simulink subsystem "Modelo_R2023b"  (R2023b)
settings: Solver=VariableStepAuto  StartTime=0.0  StopTime=10.0  RelTol=1e-3
values from neighbouring files (symbols this model uses):
  alpha_Cu = 3.9e-3    (= 0.0039)    [coeficientes.m]
  b_eq = b_m + b_l/(r_m2l^2)    (= 2.19444444444e-05)    [coeficientes.m]
  C_ts = 0.818    [coeficientes.m]
  g = 9.80665    [coeficientes.m]
  J_eq = J_m + J_l/(r_m2l^2)    (= 4.58263888889e-05)    [coeficientes.m]
  k_l = 0.1    [coeficientes.m]
  L_d = 6.6e-3    (= 0.0066)    [coeficientes.m]
  L_ls = 0.8e-3    (= 0.0008)    [coeficientes.m]
  L_q = 5.8e-3    (= 0.0058)    [coeficientes.m]
  lambda = 0.016    [coeficientes.m]
  Pp = 3    [coeficientes.m]
  r_m2l = 120.0    (= 120)    [coeficientes.m]
  R_sREF = 1.02    [coeficientes.m]
  R_tsamb = 146.7    [coeficientes.m]
  T_amb = 20    [coeficientes.m]
  T_sREF = 20    [coeficientes.m]
libraries: mcbcontrolslib x2
settings Model: Creator=barrios14101  LastModifiedBy=barrios14101
settings RTWCC: GPUComputeCapability=5.0
settings ConfigComp: CovBoundaryAbsTol=1.0e-5

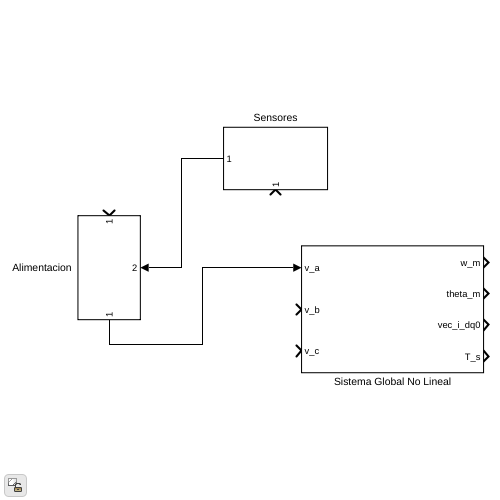
[thumbnail: Simulink's stored preview of the top-level diagram]
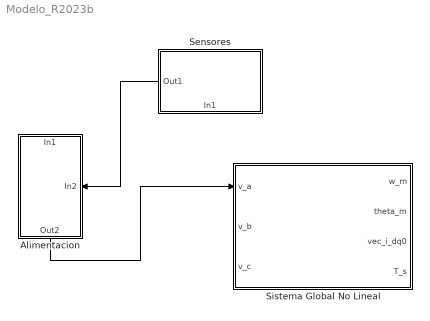
== system Modelo_R2023b ==
  Alimentacion : Subsystem
      settings: PortSchema="{\"entries\":[{\"content\":{\"sides\":[{\"content\":{\"connectorIds\":[\"In1\"]},\"type\":\"ConnectorPlacement.EquallySpacedRectSide\",\"uuid\":\"0c953847-a542-44e1-afa1-eb16e3fe163f\"},{\"content\":{\"connectorIds\":[\"Out1\"],\"side\":\"RIGHT\"},\"type\":\"ConnectorPlacement.EquallySpacedRectSide\",\"uuid\":\"d6f8d29b-16c5-463f-b013-7003ed613fe0\"},{\"content\":{\"connectorIds\":[\"In2\"],\"side\":\"TOP\"},\"type\":\"ConnectorPlacement.EquallySpacedRectSide\",\"uuid\":\"60c3fb2f-c7a9-4bb3-be2b-510700c2fe0f\"},{\"content\":{\"side\":\"BOTTOM\"},\"type\":\"ConnectorPlacement.EquallySpacedRectSide\",\"uuid\":\"5571030c-c37f-4b87-b6e8-9288f1bd1f58\"}]},\"type\":\"ConnectorPlacement.EquallySpacedConnector\",\"uuid\":\"8bfbadc8-fb17-4150-9925-c98e8d49e11f\"}],\"packageUris\":[\"http://schema.mathworks.com/mf0/Connector/R2020b\"],\"version\":\"1.0\"}"
  Sensores : Subsystem
      settings: PortSchema="{\"entries\":[{\"content\":{\"sides\":[{\"content\":{\"connectorIds\":[\"Out1\"]},\"type\":\"ConnectorPlacement.EquallySpacedRectSide\",\"uuid\":\"0c953847-a542-44e1-afa1-eb16e3fe163f\"},{\"content\":{\"side\":\"RIGHT\"},\"type\":\"ConnectorPlacement.EquallySpacedRectSide\",\"uuid\":\"d6f8d29b-16c5-463f-b013-7003ed613fe0\"},{\"content\":{\"side\":\"TOP\"},\"type\":\"ConnectorPlacement.EquallySpacedRectSide\",\"uuid\":\"60c3fb2f-c7a9-4bb3-be2b-510700c2fe0f\"},{\"content\":{\"connectorIds\":[\"In1\"],\"side\":\"BOTTOM\"},\"type\":\"ConnectorPlacement.EquallySpacedRectSide\",\"uuid\":\"48731a4e-21f3-48a9-965b-1bc0b841acdd\"}]},\"type\":\"ConnectorPlacement.EquallySpacedConnector\",\"uuid\":\"8bfbadc8-fb17-4150-9925-c98e8d49e11f\"}],\"packageUris\":[\"http://schema.mathworks.com/mf0/Connector/R2020b\"],\"version\":\"1.0\"}"
  Sistema Global No Lineal : Subsystem
  wires:
  Alimentacion/1(Out2) -> Sistema Global No Lineal/1(v_a)
  Sensores/1(Out1) -> Alimentacion/2(In2)

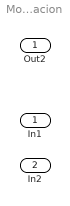
== system Modelo_R2023b/Alimentacion ==
  In1 : Inport
  In2 : Inport  Port=2
  Out2 : Outport

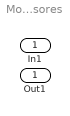
== system Modelo_R2023b/Sensores ==
  In1 : Inport
  Out1 : Outport

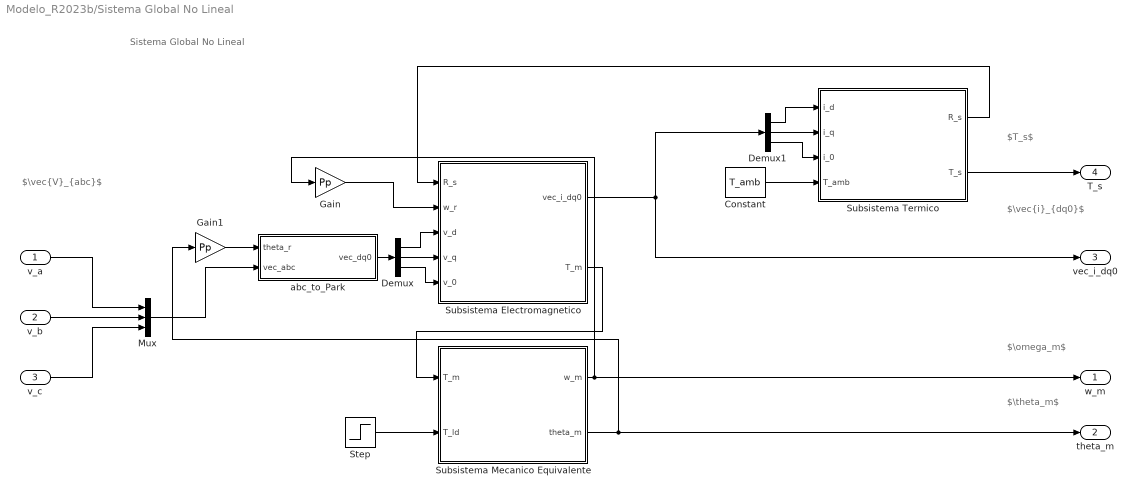
== system Modelo_R2023b/Sistema Global No Lineal ==
  note: $\omega_m$
  note: $T_s$
  note: $\vec{i}_{dq0}$
  note: $\vec{V}_{abc}$
  note: Sistema Global No Lineal
  note: $\theta_m$
  v_a : Inport
  v_b : Inport  Port=2
  v_c : Inport  Port=3
  Constant : Constant  Value=T_amb
  Demux : Demux  Outputs=3
  Demux1 : Demux  Outputs=3
  Gain : Gain  Gain=Pp
  Gain1 : Gain  Gain=Pp
  Mux : Mux  Inputs=3
  Step : Step  Time=0  After=15  SampleTime=0
  Subsistema Electromagnetico : Subsystem
  Subsistema Mecanico Equivalente : Subsystem
  Subsistema Termico : Subsystem
  abc_to_Park : Subsystem  TreatAsAtomicUnit=on
  w_m : Outport
  theta_m : Outport  Port=2
  vec_i_dq0 : Outport  Port=3
  T_s : Outport  Port=4
  wires:
  Subsistema Termico/2(T_s) -> T_s/1
  Subsistema Electromagnetico/1(vec_i_dq0) -> vec_i_dq0/1, Demux1/1
  Subsistema Mecanico Equivalente/1(w_m) -> w_m/1, Gain/1
  Subsistema Mecanico Equivalente/2(theta_m) -> theta_m/1, Gain1/1
  Subsistema Electromagnetico/2(T_m) -> Subsistema Mecanico Equivalente/1(T_m)
  Demux1/2 -> Subsistema Termico/2(i_q)
  Subsistema Termico/1(R_s) -> Subsistema Electromagnetico/1(R_s)
  abc_to_Park/1(vec_dq0) -> Demux/1
  Gain1/1 -> abc_to_Park/1(theta_r)
  Gain/1 -> Subsistema Electromagnetico/2(w_r)
  Step/1 -> Subsistema Mecanico Equivalente/2(T_ld)
  v_a/1 -> Mux/1
  Mux/1 -> abc_to_Park/2(vec_abc)
  Demux1/1 -> Subsistema Termico/1(i_d)
  v_b/1 -> Mux/2
  Demux/3 -> Subsistema Electromagnetico/5(v_0)
  Demux/2 -> Subsistema Electromagnetico/4(v_q)
  Demux/1 -> Subsistema Electromagnetico/3(v_d)
  Demux1/3 -> Subsistema Termico/3(i_0)
  v_c/1 -> Mux/3
  Constant/1 -> Subsistema Termico/4(T_amb)

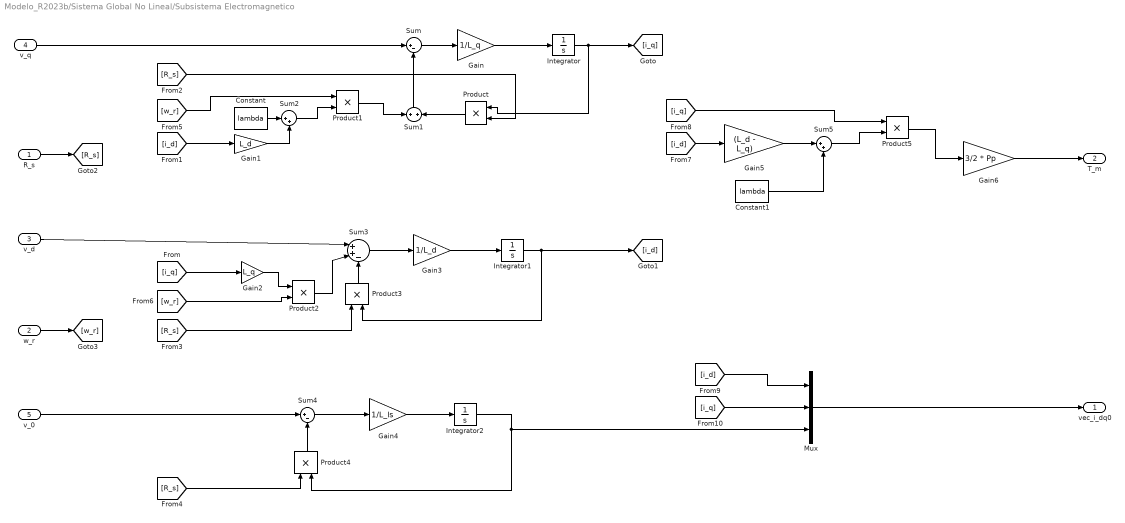
== system Modelo_R2023b/Sistema Global No Lineal/Subsistema Electromagnetico ==
  R_s : Inport
  w_r : Inport  Port=2
  v_d : Inport  Port=3
  v_q : Inport  Port=4
  v_0 : Inport  Port=5
  Constant : Constant  Value=lambda
  Constant1 : Constant  Value=lambda
  Gain : Gain  Gain=1/L_q
  Gain1 : Gain  Gain=L_d
  Gain2 : Gain  Gain=L_q
  Gain3 : Gain  Gain=1/L_d
  Gain4 : Gain  Gain=1/L_ls
  Gain5 : Gain  Gain=(L_d - L_q)
  Gain6 : Gain  Gain=3/2 * Pp
  Integrator : Integrator
  Integrator1 : Integrator
  Integrator2 : Integrator
  Mux : Mux  Inputs=3
  Product{,1..5} (6 alike) : Product
  Sum : Sum  Inputs=|+-
  Sum1 : Sum
  Sum2 : Sum  Inputs=|++
  Sum3 : Sum  Inputs=|++-
  Sum4 : Sum  Inputs=|+-
  Sum5 : Sum  Inputs=|++
  vec_i_dq0 : Outport
  T_m : Outport  Port=2
  wires:
  Gain1/1 -> Sum2/2
  Product1/1 -> Sum1/1
  Sum2/1 -> Product1/2
  Constant/1 -> Sum2/1
  Product/1 -> Sum1/2
  Sum/1 -> Gain/1
  Sum1/1 -> Sum/2
  v_q/1 -> Sum/1
  Gain/1 -> Integrator/1
  Product3/1 -> Sum3/3
  Gain3/1 -> Integrator1/1
  Sum3/1 -> Gain3/1
  Product2/1 -> Sum3/2
  Gain2/1 -> Product2/1
  v_d/1 -> Sum3/1
  Product4/1 -> Sum4/2
  Integrator2/1 -> Mux/3, Product4/2
  Gain4/1 -> Integrator2/1
  Sum4/1 -> Gain4/1
  v_0/1 -> Sum4/1
  Gain5/1 -> Sum5/1
  Sum5/1 -> Product5/2
  Integrator1/1 -> [i_d], Product3/2
  Constant1/1 -> Sum5/2
  Product5/1 -> Gain6/1
  Integrator/1 -> [i_q], Product/1
  Gain6/1 -> T_m/1
  [i_q] -> Gain2/1
  [i_d] -> Gain1/1
  [R_s] -> Product/2
  R_s/1 -> [R_s]
  [R_s] -> Product3/1
  [R_s] -> Product4/1
  w_r/1 -> [w_r]
  [w_r] -> Product1/1
  [w_r] -> Product2/2
  [i_d] -> Gain5/1
  [i_q] -> Product5/1
  [i_q] -> Mux/2
  [i_d] -> Mux/1
  Mux/1 -> vec_i_dq0/1

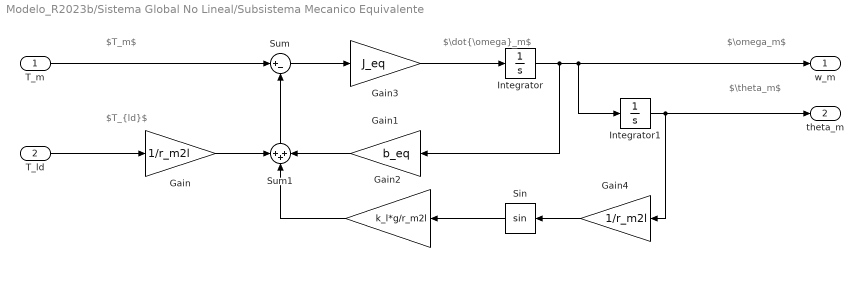
== system Modelo_R2023b/Sistema Global No Lineal/Subsistema Mecanico Equivalente ==
  note: $T_m$
  note: $T_{ld}$
  note: $\dot{\omega}_m$
  note: $\omega_m$
  note: $\theta_m$
  T_m : Inport
  T_ld : Inport  Port=2
  Gain : Gain  Gain=1/r_m2l
  Gain1 : Gain  Gain=b_eq
  Gain2 : Gain  Gain=k_l*g/r_m2l
  Gain3 : Gain  Gain=J_eq
  Gain4 : Gain  Gain=1/r_m2l
  Integrator : Integrator
  Integrator1 : Integrator
  Sin : Trigonometry
  Sum : Sum  Inputs=|+-
  Sum1 : Sum  Inputs=+++
  w_m : Outport
  theta_m : Outport  Port=2
  wires:
  Integrator/1 -> Integrator1/1, w_m/1, Gain1/1
  Integrator1/1 -> theta_m/1, Gain4/1
  Sum/1 -> Gain3/1
  T_m/1 -> Sum/1
  Sum1/1 -> Sum/2
  Gain2/1 -> Sum1/2
  Gain/1 -> Sum1/1
  Sin/1 -> Gain2/1
  Gain1/1 -> Sum1/3
  Gain3/1 -> Integrator/1
  Gain4/1 -> Sin/1
  T_ld/1 -> Gain/1

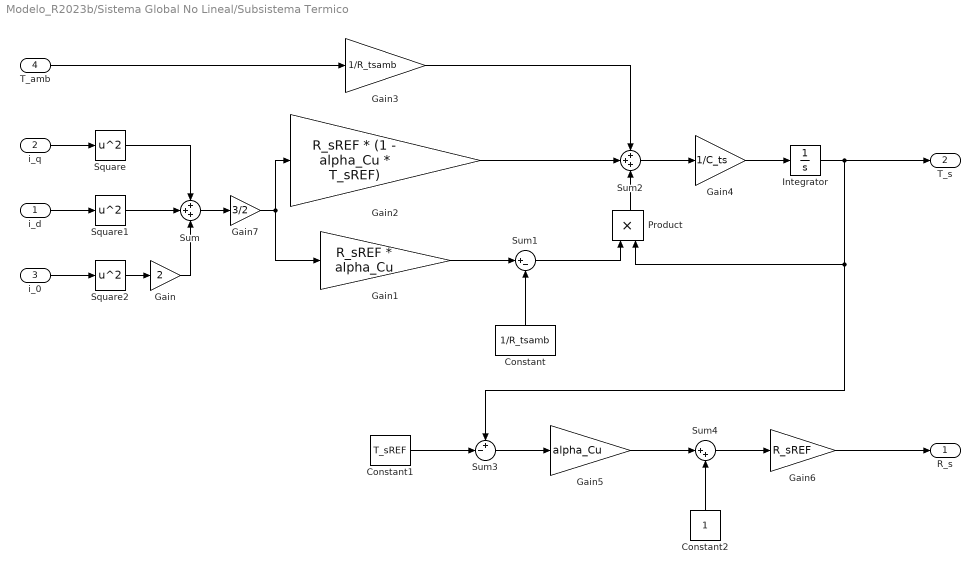
== system Modelo_R2023b/Sistema Global No Lineal/Subsistema Termico ==
  i_d : Inport
  i_q : Inport  Port=2
  i_0 : Inport  Port=3
  T_amb : Inport  Port=4
  Constant : Constant  Value=1/R_tsamb
  Constant1 : Constant  Value=T_sREF
  Constant2 : Constant
  Gain : Gain  Gain=2
  Gain1 : Gain  Gain=R_sREF * alpha_Cu
  Gain2 : Gain  Gain="R_sREF * (1 -  alpha_Cu * T_sREF)"
  Gain3 : Gain  Gain=1/R_tsamb
  Gain4 : Gain  Gain=1/C_ts
  Gain5 : Gain  Gain=alpha_Cu
  Gain6 : Gain  Gain=R_sREF
  Gain7 : Gain  Gain=3/2
  Integrator : Integrator
  Product : Product
  Square : Math  Operator=square
  Square1 : Math  Operator=square
  Square2 : Math  Operator=square
  Sum : Sum  Inputs=+++
  Sum1 : Sum  Inputs=|+-
  Sum2 : Sum  Inputs=+++
  Sum3 : Sum  Inputs=+-|
  Sum4 : Sum  Inputs=|++
  R_s : Outport
  T_s : Outport  Port=2
  wires:
  Integrator/1 -> Sum3/1, Product/2, T_s/1
  Gain6/1 -> R_s/1
  Gain7/1 -> Gain2/1, Gain1/1
  Sum4/1 -> Gain6/1
  Constant1/1 -> Sum3/2
  Gain/1 -> Sum/3
  Gain5/1 -> Sum4/1
  Gain1/1 -> Sum1/1
  Constant/1 -> Sum1/2
  Sum3/1 -> Gain5/1
  Sum1/1 -> Product/1
  T_amb/1 -> Gain3/1
  Sum/1 -> Gain7/1
  Constant2/1 -> Sum4/2
  Square2/1 -> Gain/1
  Sum2/1 -> Gain4/1
  i_0/1 -> Square2/1
  i_d/1 -> Square1/1
  Square1/1 -> Sum/2
  Square/1 -> Sum/1
  Gain2/1 -> Sum2/2
  Gain4/1 -> Integrator/1
  Product/1 -> Sum2/3
  Gain3/1 -> Sum2/1
  i_q/1 -> Square/1

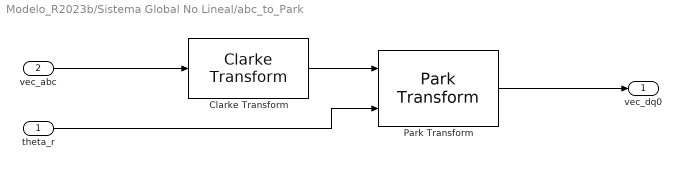
== system Modelo_R2023b/Sistema Global No Lineal/abc_to_Park ==
  theta_r : Inport
  vec_abc : Inport  Port=2
  Clarke Transform : mcbcontrolslib/Clarke Transform  VariantControl=Variant2  EnPowerInv=off  PhaseInput=Three inputs
      settings: LibrarySourceBlock=mcblib/Controls/Math Transforms/Clarke Transform
  Park Transform : mcbcontrolslib/Park Transform  AxisAlignment=D-axis  PhaseInput=Three inputs  ThetaInput=Electrical position  AngleInput=Radians  N_points=1024
      settings: LibrarySourceBlock=mcblib/Controls/Math Transforms/Park Transform
  vec_dq0 : Outport
  wires:
  theta_r/1 -> Park Transform/2
  Park Transform/1 -> vec_dq0/1
  vec_abc/1 -> Clarke Transform/1
  Clarke Transform/1 -> Park Transform/1
